simulink model "Multicopter_Testbed"  (R2012b)
settings: Solver=FixedStepDiscrete  SolverMode=SingleTasking  StartTime=0.0  StopTime=inf  FixedStep=Sampletime.Sim  MaxStep=0.005  MinStep=0.0001  RelTol=1e-5
PreLoadFcn:
  | addpath([cd filesep 'Multicopter_Simulation_Data'])
  | initMulticopterSimulationBus;
  | initOveroControlBus;
  | initMulticopterSimulation;
undefined symbols (not defined in the file): Airframe_Pelican, DiscIntNeverNeededParam, Environment_Earth, gcbh, quat_fr_euler, rad, Sampletime, Sensor_Autopilot, vrmfunc
(part 1 of 3)
settings Model: Creator=Thomas  LastModifiedBy=s0726179
settings SolverCC: InitialStep=0.001  NumberNewtonIterations=4
settings DataIOCC: SignalLoggingSaveFormat=ModelDataLogs
settings DebuggingCC: Int32ToFloatConvMsg=none  ParameterPrecisionLossMsg=none  FcnCallInpInsideContextMsg=UseLocalSettings
settings HardwareCC: ProdIntDivRoundTo=Zero  ProdEndianess=LittleEndian  ProdHWDeviceType=Generic->32-bit x86 compatible
settings ModelReferenceCC: UpdateModelReferenceTargets=Force
settings GRTTargetCC: CombineOutputUpdateFcns=off  GRTInterface=on

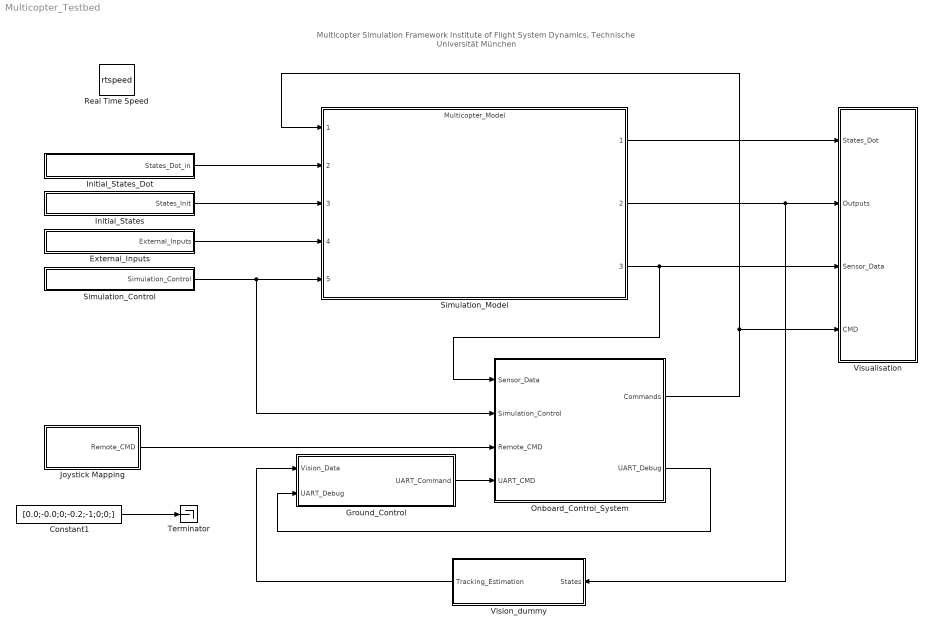
== system Multicopter_Testbed ==
  note: Multicopter Simulation Framework
      | Institute of Flight System Dynamics, Technische Universität München
  Constant1 : Constant  Value=[0.0;-0.0;0;-0.2;-1;0;0;]
  External_Inputs : Subsystem
  Ground_Control : Subsystem
  Initial_States : Subsystem
  Initial_States_Dot : Subsystem
  Joystick Mapping : Subsystem
  Onboard_Control_System : Subsystem
  Real Time Speed : S-Function  FunctionName=rtspeed  Parameters=speed  EnableBusSupport=off  mask(Simulink Realtime Synchronization){speed=1}
      mask prompts: speed "Simulation Speed (1 = realtime)"
      mask help: Slows down simulation to desired real time speed.
      mask Display:
      | ang=(0:0.0125:1)*2*pi;
      | xp=100*cos(ang);
      | yp=100*sin(ang);
      | plot(-145,-130,155,170,xp,yp,[0 0 70*sqrt(2)/2],[70 0 70*sqrt(2)/2],[-40 40 40 -40 -40],[150 150 120 120 150],[-15 -15],[120 98.5],[15 15],[120 98.5],[100*cos((45+9)/180*pi) 100*cos((45+9)/180*pi)+30 100*cos((45-9)/180*pi)+30 100*cos((45-9)/180*pi)],[100*sin((45+9)/180*pi) 100*sin((45+9)/180*pi)+30 100*sin((45-9)/180*pi)+30 100*sin((45-9)/180*pi)]);
  Simulation_Control : Subsystem
  Simulation_Model : ModelReference  ModelNameDialog=Multicopter_Model  ParameterArgumentNames=Airframe_Data,Environment_Data,Sensor_Data  ParameterArgumentValues=Airframe_Data,Environment_Data,Sensor_Data  ModelReferenceVersion=1.849  CopyOfModelName=Multicopter_Model  CopyOfModelProtected=on  DefaultDataLogging=off  mask{Airframe_Data=Airframe_Pelican, Environment_Data=Environment_Earth, Sensor_Data=Sensor_Autopilot}
  Terminator : Terminator
  Vision_dummy : Subsystem
  Visualisation : Subsystem
  wires:
  Simulation_Model/1 -> Visualisation/1(States_Dot)
  Simulation_Model/2 -> Visualisation/2(Outputs), Vision_dummy/1(States)
  Simulation_Control/1(Simulation_Control) -> Onboard_Control_System/2(Simulation_Control), Simulation_Model/5
  External_Inputs/1(External_Inputs) -> Simulation_Model/4
  Initial_States_Dot/1(States_Dot_in) -> Simulation_Model/2
  Initial_States/1(States_Init) -> Simulation_Model/3
  Onboard_Control_System/2(UART_Debug) -> Ground_Control/2(UART_Debug)
  Ground_Control/1(UART_Command) -> Onboard_Control_System/4(UART_CMD)
  Vision_dummy/1(Tracking_Estimation) -> Ground_Control/1(Vision_Data)
  Simulation_Model/3 -> Onboard_Control_System/1(Sensor_Data), Visualisation/3(Sensor_Data)
  Onboard_Control_System/1(Commands) -> Visualisation/4(CMD), Simulation_Model/1
  Joystick Mapping/1(Remote_CMD) -> Onboard_Control_System/3(Remote_CMD)
  Constant1/1 -> Terminator/1

== system Multicopter_Testbed/External_Inputs ==
  Bus Creator : BusCreator  Inputs=2  OutDataTypeStr=Bus: Static_Atmosphere_Inputs_Bus
  Bus Creator1 : BusCreator  Inputs=1  OutDataTypeStr=Bus: Dynamic_Atmosphere_Inputs_Bus
  Bus Creator2 : BusCreator  Inputs=2  OutDataTypeStr=Bus: Environment_Inputs_Bus
  Bus Creator3 : BusCreator  Inputs=2  OutDataTypeStr=Bus: External_Inputs_Bus
  Bus Creator4 : BusCreator  Inputs=2  OutDataTypeStr=Bus: Atmosphere_Inputs_Bus
  Bus Creator5 : BusCreator  Inputs=8  OutDataTypeStr=Bus: Airframe_Inputs_Bus
  Constant : Constant  Value=[0;0;0]  VectorParams1D=off
  Constant1 : Constant  Value=5  VectorParams1D=off
  Constant{4..11} (8 alike) : Constant  VectorParams1D=off
  Constant2 : Constant  Value=[0;0;0]  VectorParams1D=off
  Constant3 : Constant  Value=0  VectorParams1D=off
  External_Inputs : Outport  OutDataTypeStr=Bus: External_Inputs_Bus
  wires:
  Constant11/1 -> Bus Creator5/8  "Condition_Drive_8"
  Constant10/1 -> Bus Creator5/7  "Condition_Drive_7"
  Constant9/1 -> Bus Creator5/6  "Condition_Drive_6"
  Constant8/1 -> Bus Creator5/5  "Condition_Drive_5"
  Constant7/1 -> Bus Creator5/4  "Condition_Drive_4"
  Constant6/1 -> Bus Creator5/3  "Condition_Drive_3"
  Constant5/1 -> Bus Creator5/2  "Condition_Drive_2"
  Constant4/1 -> Bus Creator5/1  "Condition_Drive_1"
  Bus Creator5/1 -> Bus Creator3/2  "Airframe_Inputs"
  Bus Creator4/1 -> Bus Creator2/1  "Atmosphere_Inputs"
  Bus Creator3/1 -> External_Inputs/1
  Bus Creator2/1 -> Bus Creator3/1  "Environment_Inputs"
  Bus Creator1/1 -> Bus Creator4/2  "Dynamic_Atmosphere_Inputs"
  Bus Creator/1 -> Bus Creator4/1  "Static_Atmosphere_Inputs"
  Constant3/1 -> Bus Creator/2  "Delta_Pressure_MSL"
  Constant2/1 -> Bus Creator2/2  "B_Dist_R_O"
  Constant1/1 -> Bus Creator/1  "Delta_Temperature_MSL"
  Constant/1 -> Bus Creator1/1  "VEL_Wind_A_E_O"

== system Multicopter_Testbed/Ground_Control ==
  Vision_Data : Inport
  UART_Debug : Inport  Port=2
  Bus Selector : BusSelector  OutputSignals=Telemetry
  Constant1 : Constant  Value=zeros(12,1)  OutDataTypeStr=single
  Extended_Debug_Demux : Subsystem
  Rate Transition2 : RateTransition  OutPortSampleTimeOpt=Inherit
  Terminator : Terminator
  Terminator1 : Terminator
  Terminator2 : Terminator
  UART_Command : Outport
  wires:
  UART_Debug/1 -> Bus Selector/1
  Vision_Data/1 -> Rate Transition2/1
  Constant1/1 -> UART_Command/1
  Rate Transition2/1 -> Terminator2/1
  Extended_Debug_Demux/1(Quad_Data) -> Terminator1/1
  Bus Selector/1 -> Extended_Debug_Demux/1(Debug_Channels), Terminator/1  "<Telemetry>"

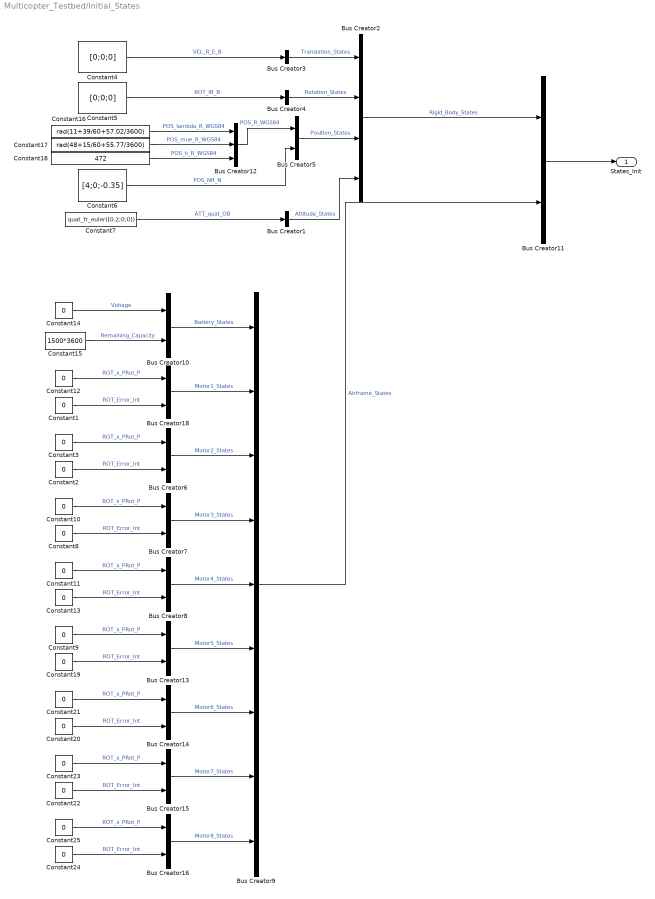
== system Multicopter_Testbed/Initial_States ==
  Bus Creator1 : BusCreator  Inputs=1  OutDataTypeStr=Bus: Attitude_States_Bus
  Bus Creator10 : BusCreator  Inputs=2  OutDataTypeStr=Bus: Battery_States_Bus
  Bus Creator11 : BusCreator  Inputs=2  OutDataTypeStr=Bus: States_Bus
  Bus Creator12 : BusCreator  Inputs=3  OutDataTypeStr=Bus: POS_R_WGS84_Bus
  Bus Creator{6..8,13..16,18} (8 alike) : BusCreator  Inputs=2  OutDataTypeStr=Bus: Motor_States_Bus
  Bus Creator2 : BusCreator  OutDataTypeStr=Bus: Rigid_Body_States_Bus
  Bus Creator3 : BusCreator  Inputs=1  OutDataTypeStr=Bus: Translation_States_Bus
  Bus Creator4 : BusCreator  Inputs=1  OutDataTypeStr=Bus: Rotation_States_Bus
  Bus Creator5 : BusCreator  Inputs=2  OutDataTypeStr=Bus: Position_States_Bus
  Bus Creator9 : BusCreator  Inputs=9  OutDataTypeStr=Bus: Airframe_States_Bus
  Constant{1..3,8..14,19..25} (17 alike) : Constant  Value=0
  Constant15 : Constant  Value=1500*3600
  Constant16 : Constant  Value=rad(11+39/60+57.02/3600)  VectorParams1D=off
  Constant17 : Constant  Value=rad(48+15/60+55.77/3600)  VectorParams1D=off
  Constant18 : Constant  Value=472  VectorParams1D=off
  Constant4 : Constant  Value=[0;0;0]  VectorParams1D=off
  Constant5 : Constant  Value=[0;0;0]  VectorParams1D=off
  Constant6 : Constant  Value=[4;0;-0.35]  VectorParams1D=off
  Constant7 : Constant  Value=quat_fr_euler([0.2;0;0])  VectorParams1D=off
  States_Init : Outport  OutDataTypeStr=Bus: States_Bus
  wires:
  Bus Creator16/1 -> Bus Creator9/9  "Motor8_States"
  Bus Creator15/1 -> Bus Creator9/8  "Motor7_States"
  Constant24/1 -> Bus Creator16/2  "ROT_Error_Int"
  Constant25/1 -> Bus Creator16/1  "ROT_x_PRot_P"
  Constant22/1 -> Bus Creator15/2  "ROT_Error_Int"
  Constant23/1 -> Bus Creator15/1  "ROT_x_PRot_P"
  Constant20/1 -> Bus Creator14/2  "ROT_Error_Int"
  Constant21/1 -> Bus Creator14/1  "ROT_x_PRot_P"
  Bus Creator14/1 -> Bus Creator9/7  "Motor6_States"
  Constant19/1 -> Bus Creator13/2  "ROT_Error_Int"
  Constant9/1 -> Bus Creator13/1  "ROT_x_PRot_P"
  Bus Creator13/1 -> Bus Creator9/6  "Motor5_States"
  Constant18/1 -> Bus Creator12/3  "POS_h_R_WGS84"
  Constant17/1 -> Bus Creator12/2  "POS_mue_R_WGS84"
  Bus Creator12/1 -> Bus Creator5/1  "POS_R_WGS84"
  Constant16/1 -> Bus Creator12/1  "POS_lambda_R_WGS84"
  Constant15/1 -> Bus Creator10/2  "Remaining_Capacity"
  Constant14/1 -> Bus Creator10/1  "Voltage"
  Bus Creator10/1 -> Bus Creator9/1  "Battery_States"
  Constant13/1 -> Bus Creator8/2  "ROT_Error_Int"
  Constant11/1 -> Bus Creator8/1  "ROT_x_PRot_P"
  Constant8/1 -> Bus Creator7/2  "ROT_Error_Int"
  Constant10/1 -> Bus Creator7/1  "ROT_x_PRot_P"
  Constant2/1 -> Bus Creator6/2  "ROT_Error_Int"
  Constant3/1 -> Bus Creator6/1  "ROT_x_PRot_P"
  Bus Creator8/1 -> Bus Creator9/5  "Motor4_States"
  Bus Creator7/1 -> Bus Creator9/4  "Motor3_States"
  Bus Creator6/1 -> Bus Creator9/3  "Motor2_States"
  Constant1/1 -> Bus Creator18/2  "ROT_Error_Int"
  Bus Creator18/1 -> Bus Creator9/2  "Motor1_States"
  Constant12/1 -> Bus Creator18/1  "ROT_x_PRot_P"
  Bus Creator9/1 -> Bus Creator11/2  "Airframe_States"
  Bus Creator11/1 -> States_Init/1
  Bus Creator2/1 -> Bus Creator11/1  "Rigid_Body_States"
  Constant7/1 -> Bus Creator1/1  "ATT_quat_OB"
  Constant6/1 -> Bus Creator5/2  "POS_NR_N"
  Constant5/1 -> Bus Creator4/1  "ROT_IB_B"
  Constant4/1 -> Bus Creator3/1  "VEL_R_E_B"
  Bus Creator1/1 -> Bus Creator2/4  "Attitude_States"
  Bus Creator3/1 -> Bus Creator2/1  "Translation_States"
  Bus Creator4/1 -> Bus Creator2/2  "Rotation_States"
  Bus Creator5/1 -> Bus Creator2/3  "Position_States"

== system Multicopter_Testbed/Initial_States_Dot ==
  Bus Creator14 : BusCreator  Inputs=1  OutDataTypeStr=Bus: States_Dot_in_Bus
  Constant11 : Constant  Value=0  VectorParams1D=off
  States_Dot_in : Outport  OutDataTypeStr=Bus: States_Dot_in_Bus
  wires:
  Constant11/1 -> Bus Creator14/1  "dummy"
  Bus Creator14/1 -> States_Dot_in/1

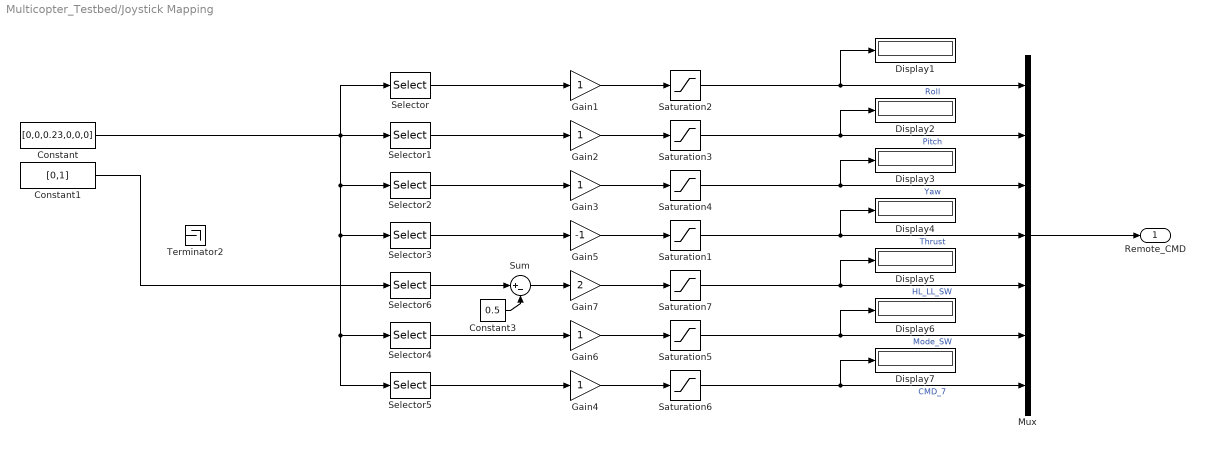
== system Multicopter_Testbed/Joystick Mapping ==
  Constant : Constant  Value=[0,0,0.23,0,0,0]
  Constant1 : Constant  Value=[0,1]
  Constant3 : Constant  Value=0.5  OutDataTypeStr=double
  Display{1..7} (7 alike) : Display
  Gain{1..4,6} (5 alike) : Gain  OutDataTypeStr=double
  Gain5 : Gain  Gain=-1  OutDataTypeStr=double
  Gain7 : Gain  Gain=2  OutDataTypeStr=double
  Mux : Mux  Inputs=7
  Saturation{1..7} (7 alike) : Saturate  UpperLimit=1  LowerLimit=-1
  Selector : Selector  IndexOptions=Index vector (dialog)  Indices=[1]  OutputSizes=1
  Selector1 : Selector  IndexOptions=Index vector (dialog)  Indices=[2]  OutputSizes=1
  Selector2 : Selector  IndexOptions=Index vector (dialog)  Indices=[6]  OutputSizes=1
  Selector3 : Selector  IndexOptions=Index vector (dialog)  Indices=[3]  OutputSizes=1
  Selector4 : Selector  IndexOptions=Index vector (dialog)  Indices=[4]  OutputSizes=1
  Selector5 : Selector  IndexOptions=Index vector (dialog)  Indices=[5]  OutputSizes=1
  Selector6 : Selector  IndexOptions=Index vector (dialog)  Indices=[2]  OutputSizes=1
  Sum : Sum  Inputs=|+-  OutDataTypeStr=double
  Terminator2 : Terminator
  Remote_CMD : Outport
  wires:
  ? -> Terminator2/1
  Constant/1 -> Selector2/1, Selector3/1, Selector5/1, Selector4/1, Selector1/1, Selector/1
  Constant1/1 -> Selector6/1
  Selector/1 -> Gain1/1
  Selector1/1 -> Gain2/1
  Selector2/1 -> Gain3/1
  Selector3/1 -> Gain5/1
  Selector4/1 -> Gain6/1
  Selector5/1 -> Gain4/1
  Selector6/1 -> Sum/1
  Sum/1 -> Gain7/1
  Constant3/1 -> Sum/2
  Gain1/1 -> Saturation2/1
  Gain2/1 -> Saturation3/1
  Gain3/1 -> Saturation4/1
  Gain5/1 -> Saturation1/1
  Gain7/1 -> Saturation7/1
  Gain6/1 -> Saturation5/1
  Gain4/1 -> Saturation6/1
  Saturation2/1 -> Mux/1, Display1/1  "Roll"
  Saturation3/1 -> Mux/2, Display2/1  "Pitch"
  Saturation4/1 -> Mux/3, Display3/1  "Yaw"
  Saturation1/1 -> Mux/4, Display4/1  "Thrust"
  Saturation7/1 -> Mux/5, Display5/1  "HL_LL_SW"
  Saturation5/1 -> Mux/6, Display6/1  "Mode_SW"
  Saturation6/1 -> Mux/7, Display7/1  "CMD_7"
  Mux/1 -> Remote_CMD/1

== system Multicopter_Testbed/Onboard_Control_System ==
  Sensor_Data : Inport  OutDataTypeStr=Bus: Sensor_Data_Bus
  Simulation_Control : Inport  Port=2  OutDataTypeStr=Bus: Simulation_Control_Bus  Interpolate=off  BusOutputAsStruct=on
  Remote_CMD : Inport  Port=3
  UART_CMD : Inport  Port=4
  LL_Pelican : Subsystem
  LL_Signal_Processing : Subsystem
  Overo_Data_Mapping : Subsystem
  Simulink_Control : Subsystem
  Commands : Outport  OutDataTypeStr=Bus: Commands_Bus
  UART_Debug : Outport  Port=2
  wires:
  LL_Pelican/1(Commands) -> Commands/1
  Sensor_Data/1 -> LL_Signal_Processing/1(Sensor_Data)
  Remote_CMD/1 -> LL_Signal_Processing/2(Remote_CMD)
  UART_CMD/1 -> Overo_Data_Mapping/1(XBee)
  LL_Signal_Processing/1(IMU_Data) -> LL_Pelican/1(IMU_Data), Simulink_Control/1(IMU)
  LL_Signal_Processing/3(Pilot_Data) -> LL_Pelican/2(Remote_CMD), Simulink_Control/3(Pilot)
  Simulink_Control/1(CMD) -> LL_Pelican/3(HL_CMD)
  LL_Signal_Processing/2(GPS_Data) -> Simulink_Control/2(GPS)
  Overo_Data_Mapping/1(Ground_Data) -> Simulink_Control/4(Data_In)
  Simulink_Control/2(Data_Out) -> UART_Debug/1
  Simulation_Control/1 -> LL_Signal_Processing/3(Simulation_Control)

== system Multicopter_Testbed/Simulation_Control ==
  Bus Creator1 : BusCreator  Inputs=2  OutDataTypeStr=Bus: State_Integration_Control_Bus
  Bus Creator2 : BusCreator  OutDataTypeStr=Bus: Simulation_Control_Bus
  Constant{1..2,4,6..7} (5 alike) : Constant  OutDataTypeStr=double
  Constant8 : Constant  Value=0  OutDataTypeStr=double
  Manual Switch : ManualSwitch  CurrentSetting=0
  Simulation_Control : Outport  OutDataTypeStr=Bus: Simulation_Control_Bus
  wires:
  Bus Creator1/1 -> Bus Creator2/1  "State_Integration_Control"
  Bus Creator2/1 -> Simulation_Control/1
  Constant8/1 -> Manual Switch/2
  Constant7/1 -> Manual Switch/1
  Manual Switch/1 -> Bus Creator1/2  "Reset"
  Constant6/1 -> Bus Creator2/4  "Translation_SW_on"
  Constant4/1 -> Bus Creator2/3  "Rotation_SW_on"
  Constant1/1 -> Bus Creator2/2  "Sensor_Errors_SW_on"
  Constant2/1 -> Bus Creator1/1  "Run"

== system Multicopter_Testbed/Vision_dummy ==
  States : Inport
  Attitude Estimation : Subsystem
  Bus Creator1 : BusCreator  Inputs=3
  Bus Selector : BusSelector  OutputSignals=States.Rigid_Body_States.Position_States.POS_NR_N,States.Rigid_Body_States.Attitude_States.ATT_quat_OB
  Position Estimation : Subsystem
  Rate Transition1 : RateTransition  OutPortSampleTime=0.04
  Rate Transition2 : RateTransition  OutPortSampleTime=0.04
  Tracking_Estimation : Outport
  wires:
  States/1 -> Bus Selector/1
  Bus Selector/1 -> Rate Transition1/1  "<POS_NR_N>"
  Bus Creator1/1 -> Tracking_Estimation/1  "Tracking"
  Bus Selector/2 -> Rate Transition2/1  "<ATT_quat_OB>"
  Position Estimation/1(Out) -> Bus Creator1/1  "POS_NR_N"
  Attitude Estimation/1(Out) -> Bus Creator1/2  "ATT_quat_OB"
  Rate Transition1/1 -> Position Estimation/1(In)
  Rate Transition2/1 -> Attitude Estimation/1(In)
  Attitude Estimation/2(Psi) -> Bus Creator1/3  "Psi"

== system Multicopter_Testbed/Visualisation ==
  States_Dot : Inport  OutDataTypeStr=Bus: States_Dot_Bus
  Outputs : Inport  Port=2  OutDataTypeStr=Bus: Outputs_Bus
  Sensor_Data : Inport  Port=3  OutDataTypeStr=Bus: Sensor_Data_Bus
  CMD : Inport  Port=4
  Atmosphere : Subsystem
  Bus Selector : BusSelector  OutputSignals=Motion_Kinematics.VEL_K_R_E_N,States.Rigid_Body_States.Rotation_States.ROT_IB_B,States.Rigid_Body_States.Position_States.POS_NR_N,States.Rigid_Body_States.Attitude_States.ATT_quat_OB,Motion_Kinematics.ATT_euler_OB
  Bus Selector2 : BusSelector  OutputSignals=Airframe.FOR_MOM_Total.FOR_T_R_B,Airframe.FOR_MOM_Total.MOM_T_R_B
  Euclidean_Norm : Subsystem
      mask help: Euclidean Norm
      mask Help: Euclidean Norm
      mask Display: disp('||.||')
  Gain6 : Gain  Gain=180/pi
  Propulsion_System : Subsystem
  Scope{1,3..4,6..7} (5 alike) : Scope
      Scope1 settings: YMin=-1.25  YMax=2  MaxDataPoints=50000000
      Scope3 settings: YMin=0  YMax=25  MaxDataPoints=500000
      Scope4 settings: SaveName=ScopeData4  MaxDataPoints=500000
      Scope6 settings: YMin=-16  YMax=6  SaveName=ScopeData6  MaxDataPoints=500000
      Scope7 settings: YMin=-0.15  YMax=0.125  SaveName=ScopeData7  MaxDataPoints=50000000
  Scope5 : Scope  NumInputPorts=3
      settings: YMin=-50~0~-180  YMax=50~15~180  SaveName=ScopeData5  MaxDataPoints=500000
  Sensors : Subsystem
  Terminator : Terminator
  VR_View : Subsystem
  wires:
  States_Dot/1 -> Terminator/1
  Outputs/1 -> Bus Selector/1, Sensors/1(States), VR_View/1(States), Bus Selector2/1, Propulsion_System/1(States), Atmosphere/1(States)
  Bus Selector/1 -> Euclidean_Norm/1(u), Scope3/1  "<VEL_K_R_E_N>"
  Bus Selector/2 -> Scope1/1  "<ROT_IB_B>"
  Bus Selector/3 -> Scope5/1  "<POS_NR_N>"
  Bus Selector/4 -> Scope4/1  "<ATT_quat_OB>"
  Bus Selector2/1 -> Scope6/1  "<FOR_T_R_B>"
  Bus Selector2/2 -> Scope7/1  "<MOM_T_R_B>"
  CMD/1 -> Propulsion_System/2(CMD)
  Euclidean_Norm/1(||u||) -> Scope5/2
  Sensor_Data/1 -> Sensors/2(Sensor_Values)
  Bus Selector/5 -> Gain6/1  "<ATT_euler_OB>"
  Gain6/1 -> Scope5/3

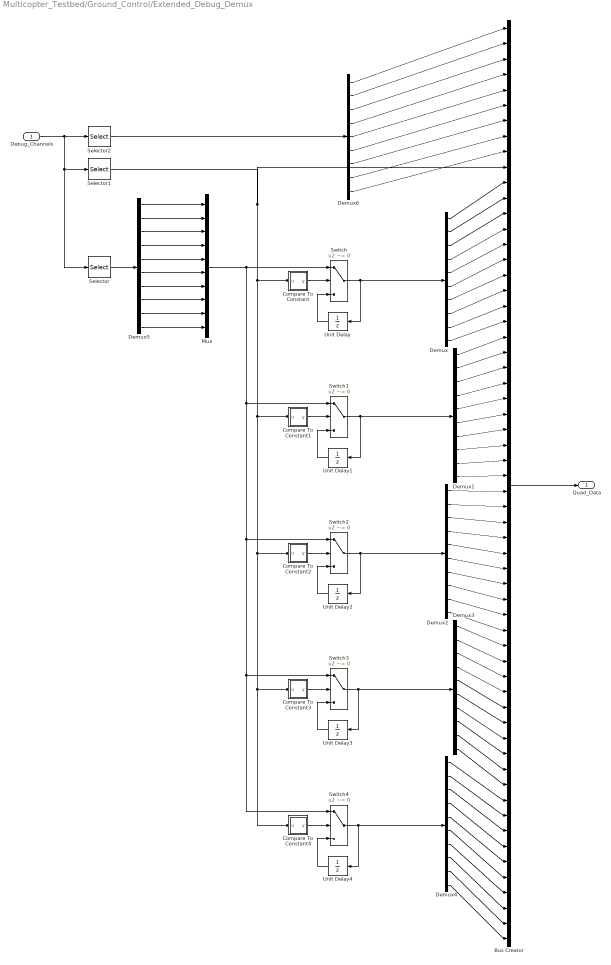
== system Multicopter_Testbed/Ground_Control/Extended_Debug_Demux ==
  Debug_Channels : Inport
  Bus Creator : BusCreator  Inputs=60
  Compare To Constant : Subsystem  mask(Compare To Constant){relop===, const=1, OutDataTypeStr=uint8, ZeroCross=off}
      mask prompts: relop "Simulink:masks:Operator_MP"; const "Simulink:masks:ConstantValue_MP"; OutDataTypeStr "Simulink:masks:OutputDataType_MP"; ZeroCross "Simulink:masks:EnableZerocrossingDetection_MP"
      mask help: Simulink:masks:CompareToConstant_MD
      mask init:
      | blkName = gcb;
      | 
      | if strcmp(get_param(gcbh,'OutDataTypeStr'),'boolean')
      | 	setValue = 'boolean';
      | else
      | 	setValue = 'fixdt(0, 8)';
      | end
      | 
      | set_param([blkName,'/Compare'],'relop',relop, ...
      | 	'OutDataTypeStr', setValue, 'ZeroCross', ZeroCross);
      | 
      | str = [relop,' C']; %default
      | 
      | const_str = get_param(blkName, 'const');
      | 
      | if isempty(strfind(const_str, ' ')) && isempty(strfind(const_str, ','))
      |     % scalar or single expression
      |     if isempty(str2num(const_str))
      |         %expression
      |         str = [relop, ' ', const_str];
      |     elseif length(const) == 1
      |         str = [relop,' ',num2str(double(const))];
      |     end
      | end
      mask TypeOptions relop: == | ~= | < | <= | >= | >
      mask TypeOptions OutDataTypeStr: Simulink:masks:uint8 | Simulink:masks:boolean
      mask Callback ZeroCross: sl('zeroCrossEnable', gcbh);
      mask Display: disp(str)
  Compare To Constant1 : Subsystem  mask(Compare To Constant){relop===, const=2, OutDataTypeStr=uint8, ZeroCross=off}
      mask prompts: relop "Simulink:masks:Operator_MP"; const "Simulink:masks:ConstantValue_MP"; OutDataTypeStr "Simulink:masks:OutputDataType_MP"; ZeroCross "Simulink:masks:EnableZerocrossingDetection_MP"
      mask help: Simulink:masks:CompareToConstant_MD
      mask init: same as Multicopter_Testbed/Ground_Control/Extended_Debug_Demux/Compare To Constant
      mask TypeOptions relop: == | ~= | < | <= | >= | >
      mask TypeOptions OutDataTypeStr: Simulink:masks:uint8 | Simulink:masks:boolean
      mask Callback ZeroCross: sl('zeroCrossEnable', gcbh);
      mask Display: disp(str)
  Compare To Constant2 : Subsystem  mask(Compare To Constant){relop===, const=3, OutDataTypeStr=uint8, ZeroCross=off}
      mask prompts: relop "Simulink:masks:Operator_MP"; const "Simulink:masks:ConstantValue_MP"; OutDataTypeStr "Simulink:masks:OutputDataType_MP"; ZeroCross "Simulink:masks:EnableZerocrossingDetection_MP"
      mask help: Simulink:masks:CompareToConstant_MD
      mask init: same as Multicopter_Testbed/Ground_Control/Extended_Debug_Demux/Compare To Constant
      mask TypeOptions relop: == | ~= | < | <= | >= | >
      mask TypeOptions OutDataTypeStr: Simulink:masks:uint8 | Simulink:masks:boolean
      mask Callback ZeroCross: sl('zeroCrossEnable', gcbh);
      mask Display: disp(str)
  Compare To Constant3 : Subsystem  mask(Compare To Constant){relop===, const=4, OutDataTypeStr=uint8, ZeroCross=off}
      mask prompts: relop "Simulink:masks:Operator_MP"; const "Simulink:masks:ConstantValue_MP"; OutDataTypeStr "Simulink:masks:OutputDataType_MP"; ZeroCross "Simulink:masks:EnableZerocrossingDetection_MP"
      mask help: Simulink:masks:CompareToConstant_MD
      mask init: same as Multicopter_Testbed/Ground_Control/Extended_Debug_Demux/Compare To Constant
      mask TypeOptions relop: == | ~= | < | <= | >= | >
      mask TypeOptions OutDataTypeStr: Simulink:masks:uint8 | Simulink:masks:boolean
      mask Callback ZeroCross: sl('zeroCrossEnable', gcbh);
      mask Display: disp(str)
  Compare To Constant4 : Subsystem  mask(Compare To Constant){relop===, const=5, OutDataTypeStr=uint8, ZeroCross=off}
      mask prompts: relop "Simulink:masks:Operator_MP"; const "Simulink:masks:ConstantValue_MP"; OutDataTypeStr "Simulink:masks:OutputDataType_MP"; ZeroCross "Simulink:masks:EnableZerocrossingDetection_MP"
      mask help: Simulink:masks:CompareToConstant_MD
      mask init: same as Multicopter_Testbed/Ground_Control/Extended_Debug_Demux/Compare To Constant
      mask TypeOptions relop: == | ~= | < | <= | >= | >
      mask TypeOptions OutDataTypeStr: Simulink:masks:uint8 | Simulink:masks:boolean
      mask Callback ZeroCross: sl('zeroCrossEnable', gcbh);
      mask Display: disp(str)
  Demux{,1..5} (6 alike) : Demux  Outputs=10
  Demux6 : Demux  Outputs=9
  Mux : Mux  Inputs=10
  Selector : Selector  InputPortWidth=20  IndexOptions=Index vector (dialog)  Indices=[11:20]  OutputSizes=1
  Selector1 : Selector  InputPortWidth=20  IndexOptions=Index vector (dialog)  Indices=[10]  OutputSizes=1
  Selector2 : Selector  InputPortWidth=20  IndexOptions=Index vector (dialog)  Indices=[1:9]  OutputSizes=1
  Switch{,1..4} (5 alike) : Switch  Criteria=u2 ~= 0
  Unit Delay{,1..4} (5 alike) : UnitDelay  SampleTime=-1
  Quad_Data : Outport
  wires:
  Debug_Channels/1 -> Selector/1, Selector1/1, Selector2/1
  Demux5/1 -> Mux/1
  Demux5/2 -> Mux/2
  Demux5/3 -> Mux/3
  Demux5/4 -> Mux/4
  Demux5/5 -> Mux/5
  Demux5/6 -> Mux/6
  Demux5/7 -> Mux/7
  Demux5/8 -> Mux/8
  Demux5/9 -> Mux/9
  Demux5/10 -> Mux/10
  Mux/1 -> Switch/1, Switch1/1, Switch2/1, Switch3/1, Switch4/1
  Demux6/1 -> Bus Creator/1
  Demux6/2 -> Bus Creator/2
  Demux6/3 -> Bus Creator/3
  Demux6/4 -> Bus Creator/4
  Demux6/5 -> Bus Creator/5
  Demux6/6 -> Bus Creator/6
  Demux6/7 -> Bus Creator/7
  Demux6/8 -> Bus Creator/8
  Demux6/9 -> Bus Creator/9
  Demux/1 -> Bus Creator/11
  Demux/2 -> Bus Creator/12
  Demux/3 -> Bus Creator/13
  Demux/4 -> Bus Creator/14
  Demux/5 -> Bus Creator/15
  Demux/6 -> Bus Creator/16
  Demux/7 -> Bus Creator/17
  Demux/8 -> Bus Creator/18
  Demux/9 -> Bus Creator/19
  Demux/10 -> Bus Creator/20
  Demux1/1 -> Bus Creator/21
  Demux1/2 -> Bus Creator/22
  Demux1/3 -> Bus Creator/23
  Demux1/4 -> Bus Creator/24
  Demux1/5 -> Bus Creator/25
  Demux1/6 -> Bus Creator/26
  Demux1/7 -> Bus Creator/27
  Demux1/8 -> Bus Creator/28
  Demux1/9 -> Bus Creator/29
  Demux1/10 -> Bus Creator/30
  Demux2/1 -> Bus Creator/31
  Demux2/2 -> Bus Creator/32
  Demux2/3 -> Bus Creator/33
  Demux2/4 -> Bus Creator/34
  Demux2/5 -> Bus Creator/35
  Demux2/6 -> Bus Creator/36
  Demux2/7 -> Bus Creator/37
  Demux2/8 -> Bus Creator/38
  Demux2/9 -> Bus Creator/39
  Demux2/10 -> Bus Creator/40
  Demux3/1 -> Bus Creator/41
  Demux3/2 -> Bus Creator/42
  Demux3/3 -> Bus Creator/43
  Demux3/4 -> Bus Creator/44
  Demux3/5 -> Bus Creator/45
  Demux3/6 -> Bus Creator/46
  Demux3/7 -> Bus Creator/47
  Demux3/8 -> Bus Creator/48
  Demux3/9 -> Bus Creator/49
  Demux3/10 -> Bus Creator/50
  Demux4/1 -> Bus Creator/51
  Demux4/2 -> Bus Creator/52
  Demux4/3 -> Bus Creator/53
  Demux4/4 -> Bus Creator/54
  Demux4/5 -> Bus Creator/55
  Demux4/6 -> Bus Creator/56
  Demux4/7 -> Bus Creator/57
  Demux4/8 -> Bus Creator/58
  Demux4/9 -> Bus Creator/59
  Demux4/10 -> Bus Creator/60
  Compare To Constant/1(y) -> Switch/2
  Switch/1 -> Demux/1, Unit Delay/1
  Unit Delay/1 -> Switch/3
  Compare To Constant1/1(y) -> Switch1/2
  Switch1/1 -> Unit Delay1/1, Demux1/1
  Unit Delay1/1 -> Switch1/3
  Compare To Constant2/1(y) -> Switch2/2
  Switch2/1 -> Unit Delay2/1, Demux2/1
  Unit Delay2/1 -> Switch2/3
  Compare To Constant3/1(y) -> Switch3/2
  Switch3/1 -> Unit Delay3/1, Demux3/1
  Unit Delay3/1 -> Switch3/3
  Compare To Constant4/1(y) -> Switch4/2
  Switch4/1 -> Unit Delay4/1, Demux4/1
  Unit Delay4/1 -> Switch4/3
  Bus Creator/1 -> Quad_Data/1
  Selector/1 -> Demux5/1
  Selector1/1 -> Compare To Constant/1(u), Compare To Constant1/1(u), Compare To Constant2/1(u), Compare To Constant3/1(u), Compare To Constant4/1(u), Bus Creator/10
  Selector2/1 -> Demux6/1

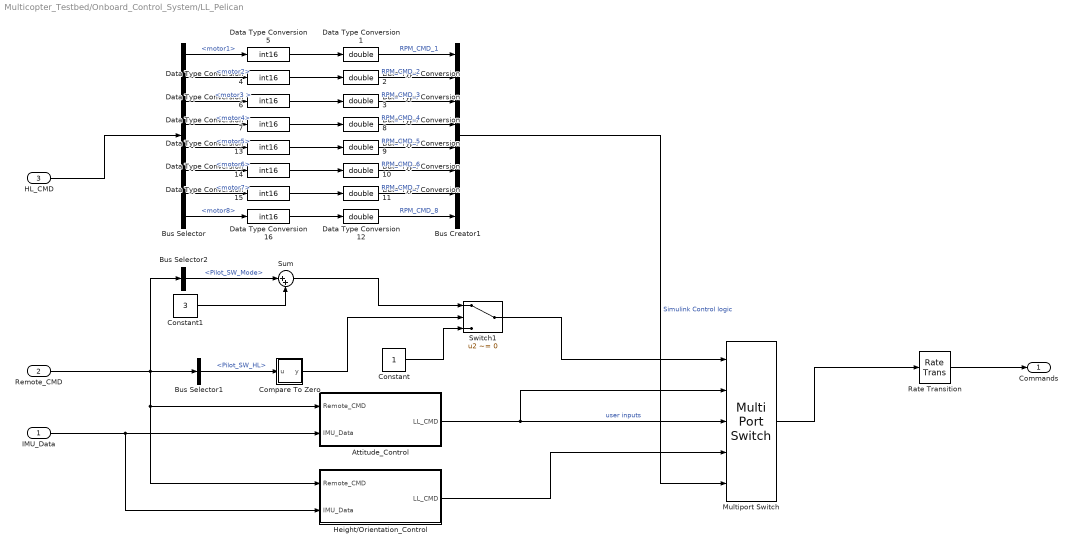
== system Multicopter_Testbed/Onboard_Control_System/LL_Pelican ==
  IMU_Data : Inport  OutDataTypeStr=Bus: FCS_IMU_Bus
  Remote_CMD : Inport  Port=2  OutDataTypeStr=Bus: FCS_Pilot_Bus
  HL_CMD : Inport  Port=3  OutDataTypeStr=Bus: FCS_CMD_Bus
  Attitude_Control : Subsystem
  Bus Creator1 : BusCreator  Inputs=8
  Bus Selector : BusSelector  OutputSignals=motor1,motor2,motor3 ,motor4,motor5,motor6,motor7,motor8
  Bus Selector1 : BusSelector  OutputSignals=Pilot_SW_HL
  Bus Selector2 : BusSelector  OutputSignals=Pilot_SW_Mode
  Compare To Zero : Subsystem  mask(Compare To Zero){relop=>, OutDataTypeStr=uint8, ZeroCross=on}
      mask prompts: relop "Simulink:masks:Operator_MP"; OutDataTypeStr "Simulink:masks:OutputDataType_MP"; ZeroCross "Simulink:masks:EnableZerocrossingDetection_MP"
      mask help: Simulink:masks:CompareToZero_MD
      mask init:
      | blkName = gcb;
      | 
      | if strcmp(get_param(gcbh,'OutDataTypeStr'),'boolean')
      | 	setValue = 'boolean';
      | else
      |     setValue = 'fixdt(0, 8)';
      | end
      | 
      | set_param([blkName,'/Compare'],'relop',relop, ...
      | 	'OutDataTypeStr', setValue, 'ZeroCross', ZeroCross);
      mask TypeOptions relop: == | ~= | < | <= | >= | >
      mask TypeOptions OutDataTypeStr: Simulink:masks:uint8 | Simulink:masks:boolean
      mask Callback ZeroCross: sl('zeroCrossEnable', gcbh);
      mask Display: disp([relop,' 0'])
  Constant : Constant
  Constant1 : Constant  Value=3  OutDataTypeStr=uint8
  Data Type Conversion{1..3,8..12} (8 alike) : DataTypeConversion  OutDataTypeStr=double
  Data Type Conversion{4..7,13..16} (8 alike) : DataTypeConversion  OutDataTypeStr=int16
  Height/Orientation_Control : Subsystem
  Multiport Switch : MultiPortSwitch  Inputs=4
  Rate Transition : RateTransition  OutPortSampleTime=Sampletime.Sim
  Sum : Sum  Inputs=|++
  Switch1 : Switch  Criteria=u2 ~= 0
  Commands : Outport  OutDataTypeStr=Bus: Commands_Bus
  wires:
  Compare To Zero/1(y) -> Switch1/2
  Attitude_Control/1(LL_CMD) -> Multiport Switch/2, Multiport Switch/3  "user inputs"
  IMU_Data/1 -> Attitude_Control/2(IMU_Data), Height/Orientation_Control/2(IMU_Data)
  Data Type Conversion12/1 -> Bus Creator1/8  "RPM_CMD_8"
  Data Type Conversion11/1 -> Bus Creator1/7  "RPM_CMD_7"
  Data Type Conversion10/1 -> Bus Creator1/6  "RPM_CMD_6"
  Data Type Conversion9/1 -> Bus Creator1/5  "RPM_CMD_5"
  Multiport Switch/1 -> Rate Transition/1
  Rate Transition/1 -> Commands/1
  Bus Selector1/1 -> Compare To Zero/1(u)  "<Pilot_SW_HL>"
  Remote_CMD/1 -> Height/Orientation_Control/1(Remote_CMD), Attitude_Control/1(Remote_CMD), Bus Selector2/1, Bus Selector1/1
  Data Type Conversion8/1 -> Bus Creator1/4  "RPM_CMD_4"
  Data Type Conversion3/1 -> Bus Creator1/3  "RPM_CMD_3"
  Data Type Conversion2/1 -> Bus Creator1/2  "RPM_CMD_2"
  Data Type Conversion1/1 -> Bus Creator1/1  "RPM_CMD_1"
  HL_CMD/1 -> Bus Selector/1
  Bus Creator1/1 -> Multiport Switch/5  "Simulink Control logic"
  Data Type Conversion5/1 -> Data Type Conversion1/1
  Bus Selector/1 -> Data Type Conversion5/1  "<motor1>"
  Bus Selector/2 -> Data Type Conversion4/1  "<motor2>"
  Bus Selector/3 -> Data Type Conversion6/1  "<motor3 >"
  Bus Selector/4 -> Data Type Conversion7/1  "<motor4>"
  Bus Selector/5 -> Data Type Conversion13/1  "<motor5>"
  Bus Selector/6 -> Data Type Conversion14/1  "<motor6>"
  Bus Selector/7 -> Data Type Conversion15/1  "<motor7>"
  Bus Selector/8 -> Data Type Conversion16/1  "<motor8>"
  Data Type Conversion4/1 -> Data Type Conversion2/1
  Data Type Conversion6/1 -> Data Type Conversion3/1
  Data Type Conversion7/1 -> Data Type Conversion8/1
  Data Type Conversion13/1 -> Data Type Conversion9/1
  Data Type Conversion14/1 -> Data Type Conversion10/1
  Data Type Conversion15/1 -> Data Type Conversion11/1
  Data Type Conversion16/1 -> Data Type Conversion12/1
  Switch1/1 -> Multiport Switch/1
  Constant/1 -> Switch1/3
  Bus Selector2/1 -> Sum/1  "<Pilot_SW_Mode>"
  Constant1/1 -> Sum/2
  Sum/1 -> Switch1/1
  Height/Orientation_Control/1(LL_CMD) -> Multiport Switch/4

== system Multicopter_Testbed/Onboard_Control_System/LL_Signal_Processing ==
  Sensor_Data : Inport  OutDataTypeStr=Bus: Sensor_Data_Bus
  Remote_CMD : Inport  Port=2
  Simulation_Control : Inport  Port=3  OutDataTypeStr=Bus: Simulation_Control_Bus  Interpolate=off  BusOutputAsStruct=on
  Bus Selector2 : BusSelector  OutputSignals=State_Integration_Control.Reset
  GPS_Signal_Processing : Subsystem
  IMU_Signal_Processing : Subsystem
  RC_Signal_Processing : Subsystem
  IMU_Data : Outport  OutDataTypeStr=Bus: FCS_IMU_Bus
  GPS_Data : Outport  Port=2  OutDataTypeStr=Bus: FCS_GPS_Bus
  Pilot_Data : Outport  Port=3  OutDataTypeStr=Bus: FCS_Pilot_Bus
  wires:
  Sensor_Data/1 -> IMU_Signal_Processing/1(Inputs), GPS_Signal_Processing/1(Inputs)
  Remote_CMD/1 -> RC_Signal_Processing/1(Remote)
  IMU_Signal_Processing/1(IMU_Data) -> IMU_Data/1
  GPS_Signal_Processing/1(GPS_Data) -> GPS_Data/1
  RC_Signal_Processing/1(RC_Data) -> Pilot_Data/1
  Simulation_Control/1 -> Bus Selector2/1
  Bus Selector2/1 -> IMU_Signal_Processing/2(Reset)  "<Reset>"

== system Multicopter_Testbed/Onboard_Control_System/Overo_Data_Mapping ==
  XBee : Inport
  Bus Creator : BusCreator  Inputs=12
  Demux : Demux  Outputs=12
  Rate Transition1 : RateTransition  Integrity=off  OutPortSampleTime=Sampletime.Onboard
  Ground_Data : Outport  OutDataTypeStr=Bus: FCS_Data_In_Bus  PortDimensions=40  SampleTime=0.001
  wires:
  Rate Transition1/1 -> Demux/1
  Bus Creator/1 -> Ground_Data/1
  Demux/12 -> Bus Creator/12  "EXT_CMD_12"
  Demux/11 -> Bus Creator/11  "EXT_CMD_11"
  Demux/10 -> Bus Creator/10  "EXT_CMD_10"
  Demux/9 -> Bus Creator/9  "EXT_CMD_9"
  Demux/8 -> Bus Creator/8  "EXT_CMD_8"
  Demux/7 -> Bus Creator/7  "EXT_CMD_7"
  Demux/6 -> Bus Creator/6  "EXT_CMD_6"
  Demux/5 -> Bus Creator/5  "EXT_CMD_5"
  Demux/4 -> Bus Creator/4  "EXT_CMD_4"
  Demux/3 -> Bus Creator/3  "EXT_CMD_3"
  Demux/2 -> Bus Creator/2  "EXT_CMD_2"
  Demux/1 -> Bus Creator/1  "EXT_CMD_1"
  XBee/1 -> Rate Transition1/1

== system Multicopter_Testbed/Onboard_Control_System/Simulink_Control ==
  note: mode_manipulator
  note: Filename: onboard_template
  IMU : Inport  OutDataTypeStr=Bus: FCS_IMU_Bus  Interpolate=off  BusOutputAsStruct=on
  GPS : Inport  Port=2  OutDataTypeStr=Bus: FCS_GPS_Bus  SampleTime=0.001  Interpolate=off  BusOutputAsStruct=on
  Pilot : Inport  Port=3  OutDataTypeStr=Bus: FCS_Pilot_Bus  Interpolate=off  BusOutputAsStruct=on
  Data_In : Inport  Port=4  OutDataTypeStr=Bus: FCS_Data_In_Bus  Interpolate=off  BusOutputAsStruct=on
  Attitude_Control : Subsystem
  Bus Creator : BusCreator  Inputs=7  OutDataTypeStr=Bus: FCS_Pilot_Bus  NonVirtualBus=on
  Bus Creator1 : BusCreator  Inputs=2  OutDataTypeStr=Bus: FCS_Data_Out_Bus  NonVirtualBus=on
  Bus Selector1 : BusSelector  OutputSignals=Pilot_Roll
  Bus Selector2 : BusSelector  OutputSignals=lambda_R_WGS84_rad
  Bus Selector3 : BusSelector  OutputSignals=EXT_CMD_1
  Bus Selector4 : BusSelector  OutputSignals=w_x_K_IB_B_radDs
  CMD_Mapping_Quadcopter : Subsystem
  Constant1 : Constant  Value=[0,0,0,-0.23]  OutDataTypeStr=single
  Constant10 : Constant  Value=zeros(20,1)  OutDataTypeStr=single
  Constant11 : Constant  OutDataTypeStr=int16
  Constant2 : Constant  Value=0  OutDataTypeStr=single
  Constant3 : Constant  Value=0  OutDataTypeStr=single
  Constant4 : Constant  Value=zeros(20,1)  OutDataTypeStr=single
  Constant5 : Constant  Value=0  OutDataTypeStr=single
  Demux : Demux
  Output_Mapping_Debug : Subsystem
  Terminator{,1..2,4..5} (5 alike) : Terminator
  CMD : Outport  OutDataTypeStr=Bus: FCS_CMD_Bus  BusOutputAsStruct=on
  Data_Out : Outport  Port=2  OutDataTypeStr=Bus: FCS_Data_Out_Bus  BusOutputAsStruct=on
  wires:
  CMD_Mapping_Quadcopter/1(HL_CMD) -> CMD/1
  GPS/1 -> Bus Selector2/1
  Bus Selector2/1 -> Terminator4/1  "<lambda_R_WGS84_rad>"
  Data_In/1 -> Bus Selector3/1
  Constant4/1 -> Bus Creator1/2  "FDR"
  Bus Selector3/1 -> Terminator5/1  "<EXT_CMD_1>"
  Bus Creator1/1 -> Data_Out/1
  Output_Mapping_Debug/1(UART_Data) -> Terminator/1
  Constant10/1 -> Bus Creator1/1  "Telemetry"
  Constant11/1 -> CMD_Mapping_Quadcopter/2(Enable_Flag)
  IMU/1 -> Attitude_Control/2(IMU), Bus Selector4/1
  Pilot/1 -> Bus Selector1/1
  Bus Selector1/1 -> Terminator2/1  "<Pilot_Roll>"
  Bus Selector4/1 -> Terminator1/1  "<w_x_K_IB_B_radDs>"
  Attitude_Control/1(RPM8) -> CMD_Mapping_Quadcopter/1(RPM8_CMD)
  Demux/1 -> Bus Creator/1  "Pilot_Roll"
  Demux/2 -> Bus Creator/2  "Pilot_Nick"
  Demux/3 -> Bus Creator/3  "Pilot_Yaw"
  Demux/4 -> Bus Creator/4  "Pilot_Thrust"
  Bus Creator/1 -> Attitude_Control/1(CMD)
  Constant2/1 -> Bus Creator/5
  Constant3/1 -> Bus Creator/6
  Constant5/1 -> Bus Creator/7
  Constant1/1 -> Demux/1

== system Multicopter_Testbed/Vision_dummy/Attitude Estimation ==
  In : Inport
  ADC1 : Subsystem  mask{resolution=0.02}
      mask prompts: resolution "Sensor resolution"
  Demux : Demux  Outputs=3
  Demux1 : Demux  Outputs=3
  Euler to Quat : Subsystem  mask(Euler angles to Quaternion){}
      mask help:
      | vector [phi; theta; psi] means:
      | 1. rotation: psi   (=eul(3)) around z axis
      | 2. rotation: theta (=eul(2)) around y axis
      | 3. rotation: phi   (=eul(1)) around x axis
      |
      | Regrettably implemented in Simulink
  Gauss Markow : Subsystem  mask(Gauss Markow){sigma=[0.05;0.05;0.05], t_corr=[0.4;0.4;0.4], T_s=0.04, dim=3}
      mask prompts: t_corr "Correlation time"; T_s "Sample time"; dim "Dimension"
      mask help: Returns a 3 dimensional vector generated by a Gauss Markow porcess.
      mask Display: disp('Gauss\nMarkow')
  Integer Delay : Delay
  Quat to Euler : Subsystem  mask(Quaternion to Euler angles){}
      mask help:
      | vector [phi; theta; psi] means:
      | 1. rotation: psi   (=eul(3)) around z axis
      | 2. rotation: theta (=eul(2)) around y axis
      | 3. rotation: phi   (=eul(1)) around x axis
  Rate Transition1 : RateTransition  OutPortSampleTime=0.04
  Saturation : Saturate  UpperLimit=pi  LowerLimit=-pi
  Saturation1 : Saturate  UpperLimit=pi/2  LowerLimit=-pi/2
  Saturation2 : Saturate  UpperLimit=pi  LowerLimit=-pi
  Sum2 : Sum  Inputs=|++
  Terminator : Terminator
  Terminator1 : Terminator
  Vector Concatenate : Concatenate  NumInputs=3  Mode=Multidimensional array
  Out : Outport
  Psi : Outport  Port=2
  wires:
  Gauss Markow/1(Noise) -> Sum2/2
  Euler to Quat/1(q) -> Integer Delay/1
  Vector Concatenate/1 -> ADC1/1(analog)
  Sum2/1 -> Demux/1
  Quat to Euler/1(euler) -> Sum2/1
  Saturation2/1 -> Vector Concatenate/3
  Demux/3 -> Saturation2/1
  Saturation1/1 -> Vector Concatenate/2
  Demux/2 -> Saturation1/1
  Saturation/1 -> Vector Concatenate/1
  Demux/1 -> Saturation/1
  In/1 -> Rate Transition1/1
  ADC1/1(digital) -> Euler to Quat/1(euler), Demux1/1
  Rate Transition1/1 -> Quat to Euler/1(q)
  Integer Delay/1 -> Out/1
  Demux1/1 -> Terminator/1
  Demux1/2 -> Terminator1/1
  Demux1/3 -> Psi/1

== system Multicopter_Testbed/Vision_dummy/Position Estimation ==
  In : Inport
  ADC1 : Subsystem  mask{resolution=0.02}
      mask prompts: resolution "Sensor resolution"
  Gauss Markow1 : Subsystem  mask(Gauss Markow){sigma=[0.05;0.05;0.05], t_corr=[0.4;0.4;0.4], T_s=0.04, dim=3}
      mask prompts: t_corr "Correlation time"; T_s "Sample time"; dim "Dimension"
      mask help: Returns a 3 dimensional vector generated by a Gauss Markow porcess.
      mask Display: disp('Gauss\nMarkow')
  Integer Delay : Delay
  Sum2 : Sum  Inputs=|++
  Out : Outport
  wires:
  Gauss Markow1/1(Noise) -> Sum2/2
  Sum2/1 -> Integer Delay/1
  ADC1/1(digital) -> Sum2/1
  In/1 -> ADC1/1(analog)
  Integer Delay/1 -> Out/1

== system Multicopter_Testbed/Visualisation/Atmosphere ==
  States : Inport
  Bus Selector4 : BusSelector  OutputSignals=Environment.Atmosphere.Static_Atmosphere.Geopotential_Height_UNIT_m,Environment.Atmosphere.Static_Atmosphere.Static_Temperature_ATM_UNIT_K,Environment.Atmosphere.Static_Atmosphere.Speed_of_Sound_ATM_UNIT_m_d_s,Environment.Atmosphere.Static_Atmosphere.Dynamic_Viscosity_ATM_UNIT_N_s_d_m2,Environment.Atmosphere.Static_Atmosphere.Kinematic_Viscosity_ATM_UNIT_m2_d_s,Environment.Atmosphere.Static_Atmosphere.Density_ATM_UNIT_kg_d_m3,Environment.Atmosphere.Static_Atmosphere.Static_Pressure_ATM_UNIT_N_d_m2,Environment.Atmosphere.Static_Atmosphere.VALID_Atmosphere_Layer
  Data Type Conversion : DataTypeConversion  OutDataTypeStr=double
  Display : Display
  Mux : Mux  Inputs=8
  wires:
  Bus Selector4/1 -> Mux/1  "<Geopotential_Height_UNIT_m>"
  Bus Selector4/2 -> Mux/2  "<Static_Temperature_ATM_UNIT_K>"
  Bus Selector4/3 -> Mux/3  "<Speed_of_Sound_ATM_UNIT_m_d_s>"
  Bus Selector4/5 -> Mux/5  "<Kinematic_Viscosity_ATM_UNIT_m2_d_s>"
  Bus Selector4/6 -> Mux/6  "<Density_ATM_UNIT_kg_d_m3>"
  Bus Selector4/7 -> Mux/7  "<Static_Pressure_ATM_UNIT_N_d_m2>"
  Bus Selector4/8 -> Data Type Conversion/1  "<VALID_Atmosphere_Layer>"
  Mux/1 -> Display/1
  Bus Selector4/4 -> Mux/4  "<Dynamic_Viscosity_ATM_UNIT_N_s_d_m2>"
  Data Type Conversion/1 -> Mux/8
  States/1 -> Bus Selector4/1

== system Multicopter_Testbed/Visualisation/Euclidean_Norm ==
  u : Inport
  Math Function : Math  Operator=square  SaturateOnIntegerOverflow=on
  Sqrt : Sqrt  SaturateOnIntegerOverflow=on
  Sum of Elements : Sum  Inputs=+
  ||u|| : Outport
  wires:
  u/1 -> Math Function/1
  Math Function/1 -> Sum of Elements/1
  Sum of Elements/1 -> Sqrt/1
  Sqrt/1 -> ||u||/1

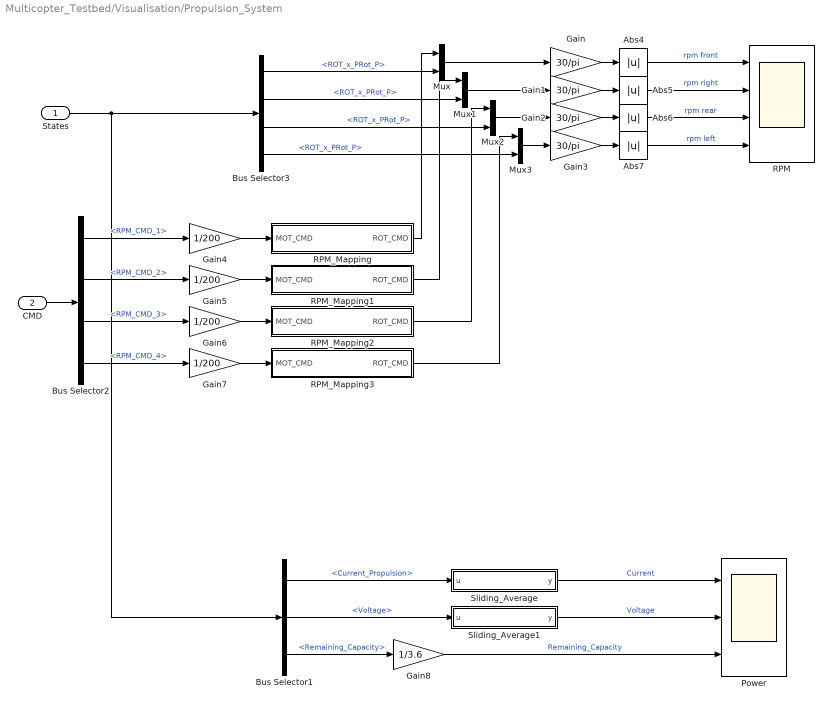
== system Multicopter_Testbed/Visualisation/Propulsion_System ==
  States : Inport
  CMD : Inport  Port=2
  Abs{4..7} (4 alike) : Abs
  Bus Selector1 : BusSelector  OutputSignals=Airframe.Current_Propulsion,States.Airframe_States.Battery_States.Voltage,States.Airframe_States.Battery_States.Remaining_Capacity
  Bus Selector2 : BusSelector  OutputSignals=RPM_CMD_1,RPM_CMD_2,RPM_CMD_3,RPM_CMD_4
  Bus Selector3 : BusSelector  OutputSignals=States.Airframe_States.Motor1_States.ROT_x_PRot_P,States.Airframe_States.Motor2_States.ROT_x_PRot_P,States.Airframe_States.Motor3_States.ROT_x_PRot_P,States.Airframe_States.Motor4_States.ROT_x_PRot_P
  Gain{,1..3} (4 alike) : Gain  Gain=30/pi
  Gain{4..7} (4 alike) : Gain  Gain=1/200
  Gain8 : Gain  Gain=1/3.6
  Mux{,1..3} (4 alike) : Mux  Inputs=2
  Power : Scope  NumInputPorts=3
      settings: TimeRange=5  YMin=0~0~0  YMax=40~12~2200  SaveName=ScopeData10  MaxDataPoints=500000
  RPM : Scope  NumInputPorts=4
      settings: TimeRange=5  YMin=500~500~500~500  YMax=9000~9000~9000~9000  SaveName=ScopeData8  MaxDataPoints=500000
  RPM_Mapping : Subsystem  mask{n_max=8980, n_min=1160}
      mask prompts: n_max "Upper RPM Limit"; n_min "Lower RPM Limit"
  RPM_Mapping1 : Subsystem  mask{n_max=8980, n_min=1160}
      mask prompts: n_max "Upper RPM Limit"; n_min "Lower RPM Limit"
  RPM_Mapping2 : Subsystem  mask{n_max=8980, n_min=1160}
      mask prompts: n_max "Upper RPM Limit"; n_min "Lower RPM Limit"
  RPM_Mapping3 : Subsystem  mask{n_max=8980, n_min=1160}
      mask prompts: n_max "Upper RPM Limit"; n_min "Lower RPM Limit"
  Sliding_Average : Subsystem
  Sliding_Average1 : Subsystem
  wires:
  Bus Selector3/3 -> Mux2/2  "<ROT_x_PRot_P>"
  Bus Selector3/4 -> Mux3/2  "<ROT_x_PRot_P>"
  Gain/1 -> Abs4/1
  Gain1/1 -> Abs5/1
  Gain2/1 -> Abs6/1
  Gain3/1 -> Abs7/1
  States/1 -> Bus Selector3/1, Bus Selector1/1
  Bus Selector1/1 -> Sliding_Average/1(u)  "<Current_Propulsion>"
  Abs4/1 -> RPM/1  "rpm front"
  Abs5/1 -> RPM/2  "rpm right"
  Abs6/1 -> RPM/3  "rpm rear"
  Abs7/1 -> RPM/4  "rpm left"
  CMD/1 -> Bus Selector2/1
  Bus Selector2/1 -> Gain4/1  "<RPM_CMD_1>"
  Bus Selector2/2 -> Gain5/1  "<RPM_CMD_2>"
  Bus Selector2/3 -> Gain6/1  "<RPM_CMD_3>"
  Bus Selector2/4 -> Gain7/1  "<RPM_CMD_4>"
  Mux/1 -> Gain/1
  Mux1/1 -> Gain1/1
  Mux2/1 -> Gain2/1
  Mux3/1 -> Gain3/1
  Bus Selector3/1 -> Mux/2  "<ROT_x_PRot_P>"
  Bus Selector3/2 -> Mux1/2  "<ROT_x_PRot_P>"
  RPM_Mapping/1(ROT_CMD) -> Mux/1
  RPM_Mapping1/1(ROT_CMD) -> Mux1/1
  RPM_Mapping2/1(ROT_CMD) -> Mux2/1
  RPM_Mapping3/1(ROT_CMD) -> Mux3/1
  Gain4/1 -> RPM_Mapping/1(MOT_CMD)
  Gain5/1 -> RPM_Mapping1/1(MOT_CMD)
  Gain6/1 -> RPM_Mapping2/1(MOT_CMD)
  Gain7/1 -> RPM_Mapping3/1(MOT_CMD)
  Bus Selector1/2 -> Sliding_Average1/1(u)  "<Voltage>"
  Bus Selector1/3 -> Gain8/1  "<Remaining_Capacity>"
  Gain8/1 -> Power/3  "Remaining_Capacity"
  Sliding_Average/1(y) -> Power/1  "Current"
  Sliding_Average1/1(y) -> Power/2  "Voltage"

== system Multicopter_Testbed/Visualisation/Sensors ==
  States : Inport
  Sensor_Values : Inport  Port=2
  Bus Selector3 : BusSelector  OutputSignals=f_R_B,ROT_IB_B,MAG_R_B,Static_Pressure_ATM,Static_Temperature_ATM,GPS_Data.POS_lambda_WGS84,GPS_Data.POS_mue_WGS84,GPS_Data.POS_h_WGS84,GPS_Data.VEL_x_E_O,GPS_Data.VEL_y_E_O,GPS_Data.VEL_z_E_O
  Bus Selector6 : BusSelector  OutputSignals=States.Rigid_Body_States.Position_States.POS_R_WGS84.POS_lambda_R_WGS84,States.Rigid_Body_States.Position_States.POS_R_WGS84.POS_mue_R_WGS84,States.Rigid_Body_States.Position_States.POS_R_WGS84.POS_h_R_WGS84
  Compare Mix1 : Subsystem
  Display : Display
      settings: Decimation=1000
  Gain3 : Gain  Gain=180/pi
  Gain4 : Gain  Gain=180/pi
  Mux : Mux  Inputs=3
  Mux1 : Mux  Inputs=3
  Scope{1..4,8} (5 alike) : Scope
      Scope1 settings: YMin=-1.5e-005  YMax=6e-005  MaxDataPoints=500000
      Scope2 settings: YMin=-9  YMax=4  MaxDataPoints=500000
      Scope3 settings: YMin=-25  YMax=2.5  SaveName=ScopeData3  MaxDataPoints=5000000
      Scope4 settings: YMin=-9  YMax=4  SaveName=ScopeData2  MaxDataPoints=500000
      Scope8 settings: YMin=-0.35  YMax=0.35  SaveName=ScopeData9  MaxDataPoints=500000
  Scope10 : Scope  NumInputPorts=3
      settings: YMin=0~0~0  YMax=12~50~500  SaveName=ScopeData12  MaxDataPoints=500000
  Scope9 : Scope  NumInputPorts=3
      settings: YMin=-0.7~-4~-0.9  YMax=0.3~0.5~0.5  SaveName=ScopeData11  MaxDataPoints=500000
  wires:
  States/1 -> Bus Selector6/1
  Sensor_Values/1 -> Bus Selector3/1
  Bus Selector6/1 -> Mux/1  "<POS_lambda_R_WGS84>"
  Bus Selector6/2 -> Mux/2  "<POS_mue_R_WGS84>"
  Bus Selector6/3 -> Mux/3  "<POS_h_R_WGS84>"
  Mux/1 -> Display/1, Compare Mix1/1(u1)
  Bus Selector3/9 -> Scope9/1  "<VEL_x_E_O>"
  Bus Selector3/10 -> Scope9/2  "<VEL_y_E_O>"
  Bus Selector3/11 -> Scope9/3  "<VEL_z_E_O>"
  Bus Selector3/7 -> Mux1/2  "<POS_mue_WGS84>"
  Bus Selector3/6 -> Mux1/1  "<POS_lambda_WGS84>"
  Bus Selector3/8 -> Mux1/3  "<POS_h_WGS84>"
  Mux1/1 -> Compare Mix1/2(u2)
  Compare Mix1/1(y1) -> Gain3/1
  Compare Mix1/2(y2) -> Gain4/1
  Compare Mix1/3(y3) -> Scope10/3
  Gain3/1 -> Scope10/1
  Gain4/1 -> Scope10/2
  Bus Selector3/1 -> Scope3/1  "<f_R_B>"
  Bus Selector3/2 -> Scope8/1  "<ROT_IB_B>"
  Bus Selector3/3 -> Scope1/1  "<MAG_R_B>"
  Bus Selector3/4 -> Scope2/1  "<Static_Pressure_ATM>"
  Bus Selector3/5 -> Scope4/1  "<Static_Temperature_ATM>"

== system Multicopter_Testbed/Visualisation/VR_View ==
  States : Inport
  Bus Selector1 : BusSelector  OutputSignals=States.Rigid_Body_States.Position_States.POS_NR_N,States.Rigid_Body_States.Attitude_States.ATT_quat_OB
  Constant : Constant  Value=[5;3; -1.5]  VectorParams1D=off
  Firefly_VR : S-Function  InstantiateOnLoad=on  LoadFcn=vrmfunc('FnLoad', gcbh);  InitFcn=vrmfunc('FnInit', gcbh);  StartFcn=vrmfunc('FnSimStatus', gcbh, 'running')  StopFcn=vrmfunc('FnStop', gcbh)  FunctionName=vrsfunc  Parameters=SampleTime, VideoDimensions, 0  EnableBusSupport=off  mask(Virtual Reality Sink){SampleTime=0.04, ViewEnable=on, RemoteChange=off, RemoteView=off, FieldsWritten=VW_Standing.orientation.4.1.1.double#VW_Standing.position.3.1.1.double#Firefly_group.translation.3.1.1.double#Firefly.rotation.4.1.1.double, WorldFileName=Firefly.wrl, WorldDescription=VR Plane Take-Off - Ancient Overhaul, AutoView=off, VideoDimensions=[], AllowVariableSize=off, FigureProperties=}
      mask prompts: SampleTime "Sample Time"; ViewEnable "View"; RemoteChange "Remote Change"; RemoteView "Remote View"; FieldsWritten "Fields Written"; WorldFileName "World File Name"; WorldDescription "World Description"; VideoDimensions "Video Dimensions"; AllowVariableSize "Allow Variable Size"; FigureProperties "Figure Properties"
      mask help: Controls the selected fields of a virtual world according to given inputs.
      mask init:
      | set_param(gcbh, 'MaskDisplay', vrmfunc('FnIcon'));
      settings: CopyFcn=vrmfunc('FnCopy', gcbh);  DeleteFcn=vrmfunc('FnDelete', gcbh);  PreSaveFcn=vrmfunc('FnPreSave', gcbh);  PauseFcn=vrmfunc('FnSimStatus', gcbh, 'paused');  ContinueFcn=vrmfunc('FnSimStatus', gcbh, 'running');  DestroyFcn=vrmfunc('FnDestroy', gcbh);  OpenFcn=vrmfunc('FnOpen', gcbh);  CloseFcn=vrmfunc('FnClose', gcbh);
      mask Help: helpview(vrmfunc('FnHelpTopic'), 'vr_vrsink');
      mask Display:
      | image(imread('vrblockicon.png'));
      | port_label('input', 1, 'VW_Standing.orientation');
      | port_label('input', 2, 'VW_Standing.position');
      | port_label('input', 3, 'Firefly_group.translation');
      | port_label('input', 4, 'Firefly.rotation');
  Hummingbird_VR : S-Function  InstantiateOnLoad=on  LoadFcn=vrmfunc('FnLoad', gcbh);  InitFcn=vrmfunc('FnInit', gcbh);  StartFcn=vrmfunc('FnSimStatus', gcbh, 'running')  StopFcn=vrmfunc('FnStop', gcbh)  FunctionName=vrsfunc  Parameters=SampleTime, VideoDimensions, 0  EnableBusSupport=off  mask(Virtual Reality Sink){SampleTime=0.04, ViewEnable=on, RemoteChange=off, RemoteView=on, FieldsWritten=VW_Standing.orientation.4.1.1.double#VW_Standing.position.3.1.1.double#Quad_group.translation.3.1.1.double#Quad.rotation.4.1.1.double, WorldFileName=Hummingbird.wrl, WorldDescription=Hummingbird - Field, AutoView=off, VideoDimensions=[], AllowVariableSize=off, FigureProperties=}
      mask prompts: SampleTime "Sample Time"; ViewEnable "View"; RemoteChange "Remote Change"; RemoteView "Remote View"; FieldsWritten "Fields Written"; WorldFileName "World File Name"; WorldDescription "World Description"; VideoDimensions "Video Dimensions"; AllowVariableSize "Allow Variable Size"; FigureProperties "Figure Properties"
      mask help: Controls the selected fields of a virtual world according to given inputs.
      mask init:
      | set_param(gcbh, 'MaskDisplay', vrmfunc('FnIcon'));
      settings: CopyFcn=vrmfunc('FnCopy', gcbh);  DeleteFcn=vrmfunc('FnDelete', gcbh);  PreSaveFcn=vrmfunc('FnPreSave', gcbh);  PauseFcn=vrmfunc('FnSimStatus', gcbh, 'paused');  ContinueFcn=vrmfunc('FnSimStatus', gcbh, 'running');  DestroyFcn=vrmfunc('FnDestroy', gcbh);  OpenFcn=vrmfunc('FnOpen', gcbh);  CloseFcn=vrmfunc('FnClose', gcbh);
      mask Help: helpview(vrmfunc('FnHelpTopic'), 'vr_vrsink');
      mask Display:
      | image(imread('vrblockicon.png'));
      | port_label('input', 1, 'VW_Standing.orientation');
      | port_label('input', 2, 'VW_Standing.position');
      | port_label('input', 3, 'Quad_group.translation');
      | port_label('input', 4, 'Quad.rotation');
  Quad States to VR_Inputs : Subsystem
  Rate Transition3 : RateTransition  OutPortSampleTime=0.04
  wires:
  Constant/1 -> Quad States to VR_Inputs/3(Viewer_Pos)
  Bus Selector1/1 -> Quad States to VR_Inputs/1(Quad_Pos)  "<POS_NR_N>"
  Bus Selector1/2 -> Quad States to VR_Inputs/2(Quad_Att_quat)  "<ATT_quat_OB>"
  Rate Transition3/1 -> Bus Selector1/1
  States/1 -> Rate Transition3/1
  Quad States to VR_Inputs/1(VR_VW_Att) -> Hummingbird_VR/1, Firefly_VR/1
  Quad States to VR_Inputs/2(VR_VW_Pos) -> Hummingbird_VR/2, Firefly_VR/2
  Quad States to VR_Inputs/3(VR_Quad_Pos) -> Hummingbird_VR/3, Firefly_VR/3
  Quad States to VR_Inputs/4(VR_Quad_Att) -> Hummingbird_VR/4, Firefly_VR/4

== system Multicopter_Testbed/Ground_Control/Extended_Debug_Demux/Compare To Constant ==
  u : Inport
  Compare : RelationalOperator  Operator===  OutDataTypeStr=fixdt(0, 8)  ZeroCross=off  InputSameDT=on
  Constant : Constant  DisableCoverage=on  Value=const  OutDataTypeStr=Inherit: Inherit via back propagation
  y : Outport
  wires:
  u/1 -> Compare/1
  Constant/1 -> Compare/2
  Compare/1 -> y/1

== system Multicopter_Testbed/Ground_Control/Extended_Debug_Demux/Compare To Constant1 ==
  u : Inport
  Compare : RelationalOperator  Operator===  OutDataTypeStr=fixdt(0, 8)  ZeroCross=off  InputSameDT=on
  Constant : Constant  DisableCoverage=on  Value=const  OutDataTypeStr=Inherit: Inherit via back propagation
  y : Outport
  wires:
  u/1 -> Compare/1
  Constant/1 -> Compare/2
  Compare/1 -> y/1

== system Multicopter_Testbed/Ground_Control/Extended_Debug_Demux/Compare To Constant2 ==
  u : Inport
  Compare : RelationalOperator  Operator===  OutDataTypeStr=fixdt(0, 8)  ZeroCross=off  InputSameDT=on
  Constant : Constant  DisableCoverage=on  Value=const  OutDataTypeStr=Inherit: Inherit via back propagation
  y : Outport
  wires:
  u/1 -> Compare/1
  Constant/1 -> Compare/2
  Compare/1 -> y/1

== system Multicopter_Testbed/Ground_Control/Extended_Debug_Demux/Compare To Constant3 ==
  u : Inport
  Compare : RelationalOperator  Operator===  OutDataTypeStr=fixdt(0, 8)  ZeroCross=off  InputSameDT=on
  Constant : Constant  DisableCoverage=on  Value=const  OutDataTypeStr=Inherit: Inherit via back propagation
  y : Outport
  wires:
  u/1 -> Compare/1
  Constant/1 -> Compare/2
  Compare/1 -> y/1
